simulink model "Quadcopter"  (R2022a)
settings: Solver=VariableStepAuto  StartTime=0.0  StopTime=10.0  RelTol=1e-3
settings Model: Creator=Erfan  LastModifiedBy=Erfan

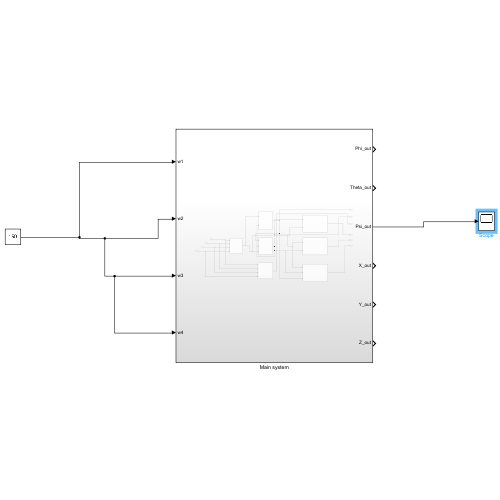
[thumbnail: Simulink's stored preview of the top-level diagram]
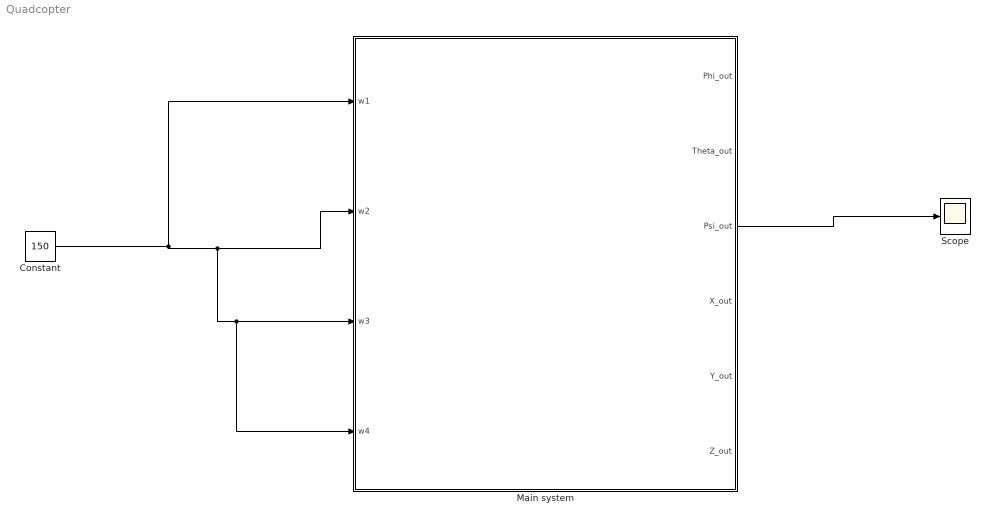
== system Quadcopter ==
  Constant : Constant  Value=150
  Main system : Subsystem
  Scope : Scope
  wires:
  Constant/1 -> Main system/4(w4), Main system/3(w3), Main system/2(w2), Main system/1(w1)
  Main system/3(Psi_out) -> Scope/1

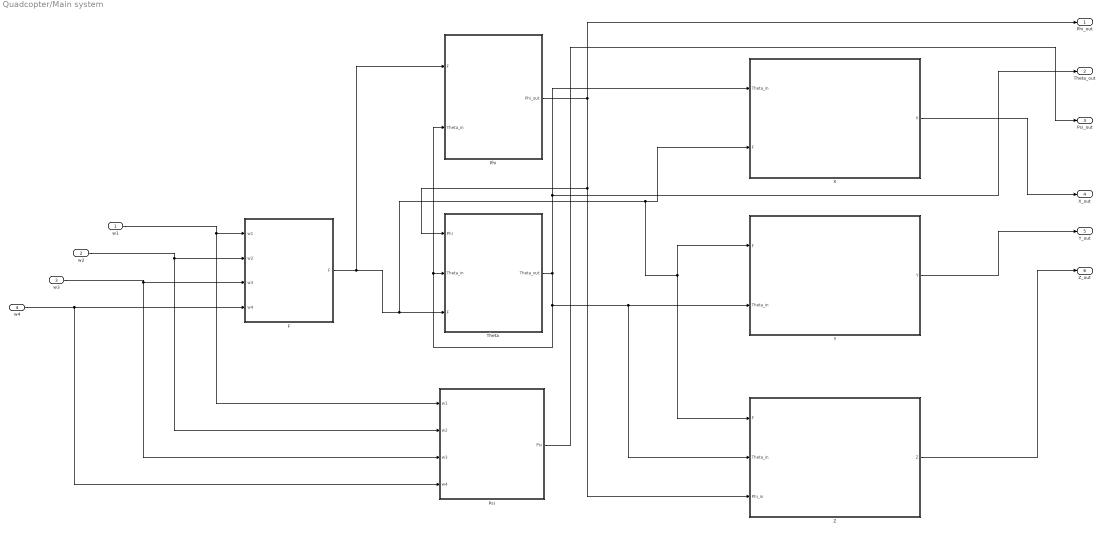
== system Quadcopter/Main system ==
  w1 : Inport
  w2 : Inport  Port=2
  w3 : Inport  Port=3
  w4 : Inport  Port=4
  F : Subsystem
  Phi : Subsystem
  Psi : Subsystem
  Theta : Subsystem
  X : Subsystem
  Y : Subsystem
  Z : Subsystem
  Phi_out : Outport
  Theta_out : Outport  Port=2
  Psi_out : Outport  Port=3
  X_out : Outport  Port=4
  Y_out : Outport  Port=5
  Z_out : Outport  Port=6
  wires:
  w1/1 -> Psi/1(w1), F/1(w1)
  w2/1 -> Psi/2(w2), F/2(w2)
  w3/1 -> Psi/3(w3), F/3(w3)
  w4/1 -> Psi/4(w4), F/4(w4)
  Phi/1(Phi_out) -> Phi_out/1, Theta/1(Phi), Z/3(Phi_in)
  F/1(F) -> Phi/1(F), Z/1(F), Y/1(F), X/2(F), Theta/3(F)
  Theta/1(Theta_out) -> Z/2(Theta_in), Y/2(Theta_in), Phi/2(Theta_in), Theta/2(Theta_in), Theta_out/1, X/1(Theta_in)
  X/1(X) -> X_out/1
  Psi/1(Psi) -> Psi_out/1
  Y/1(Y) -> Y_out/1
  Z/1(Z) -> Z_out/1

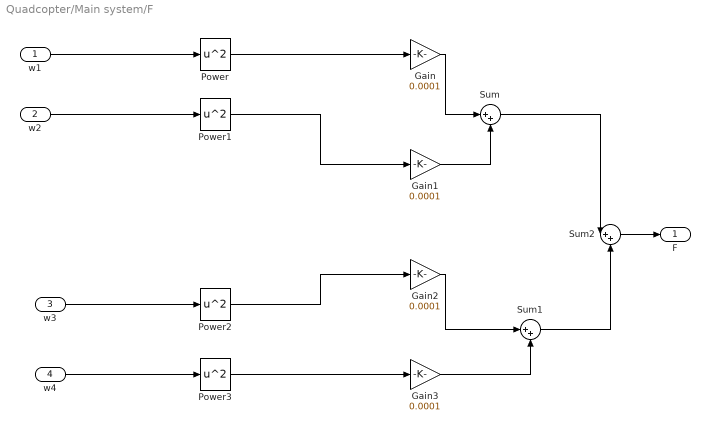
== system Quadcopter/Main system/F ==
  w1 : Inport
  w2 : Inport  Port=2
  w3 : Inport  Port=3
  w4 : Inport  Port=4
  Gain{,1..3} (4 alike) : Gain  Gain=0.0001
  Power{,1..3} (4 alike) : Math  Operator=square
  Sum : Sum  Inputs=|++
  Sum1 : Sum  Inputs=|++
  Sum2 : Sum  Inputs=|++
  F : Outport
  wires:
  Gain/1 -> Sum/1
  Sum2/1 -> F/1
  Power1/1 -> Gain1/1
  Sum/1 -> Sum2/1
  Sum1/1 -> Sum2/2
  Gain2/1 -> Sum1/1
  Power3/1 -> Gain3/1
  Gain3/1 -> Sum1/2
  Power/1 -> Gain/1
  w3/1 -> Power2/1
  w4/1 -> Power3/1
  Power2/1 -> Gain2/1
  Gain1/1 -> Sum/2
  w2/1 -> Power1/1
  w1/1 -> Power/1

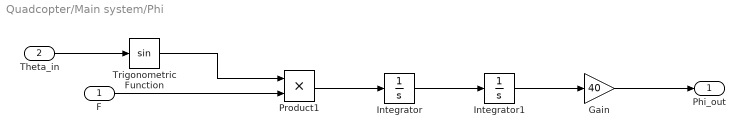
== system Quadcopter/Main system/Phi ==
  F : Inport
  Theta_in : Inport  Port=2
  Gain : Gain  Gain=40
  Integrator : Integrator
  Integrator1 : Integrator
  Product1 : Product
  Trigonometric Function : Trigonometry
  Phi_out : Outport
  wires:
  Integrator/1 -> Integrator1/1
  Gain/1 -> Phi_out/1
  Theta_in/1 -> Trigonometric Function/1
  Product1/1 -> Integrator/1
  Integrator1/1 -> Gain/1
  Trigonometric Function/1 -> Product1/1
  F/1 -> Product1/2

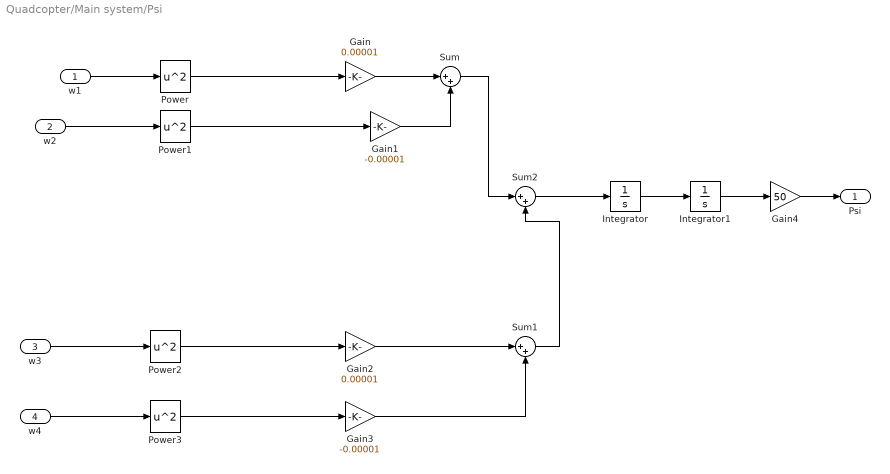
== system Quadcopter/Main system/Psi ==
  w1 : Inport
  w2 : Inport  Port=2
  w3 : Inport  Port=3
  w4 : Inport  Port=4
  Gain : Gain  Gain=0.00001
  Gain1 : Gain  Gain=-0.00001
  Gain2 : Gain  Gain=0.00001
  Gain3 : Gain  Gain=-0.00001
  Gain4 : Gain  Gain=50
  Integrator : Integrator
  Integrator1 : Integrator
  Power{,1..3} (4 alike) : Math  Operator=square
  Sum : Sum  Inputs=|++
  Sum1 : Sum  Inputs=|++
  Sum2 : Sum  Inputs=|++
  Psi : Outport
  wires:
  Power3/1 -> Gain3/1
  Power1/1 -> Gain1/1
  Gain4/1 -> Psi/1
  Gain2/1 -> Sum1/1
  Integrator1/1 -> Gain4/1
  Sum2/1 -> Integrator/1
  Sum1/1 -> Sum2/2
  Integrator/1 -> Integrator1/1
  Power/1 -> Gain/1
  Gain1/1 -> Sum/2
  Gain3/1 -> Sum1/2
  Power2/1 -> Gain2/1
  Sum/1 -> Sum2/1
  Gain/1 -> Sum/1
  w4/1 -> Power3/1
  w3/1 -> Power2/1
  w2/1 -> Power1/1
  w1/1 -> Power/1

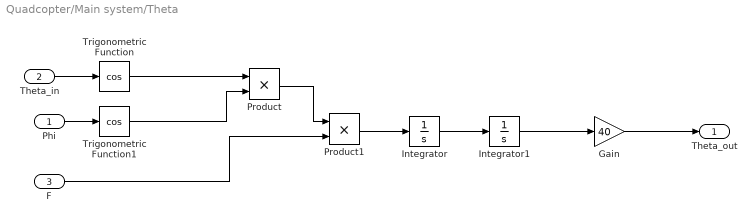
== system Quadcopter/Main system/Theta ==
  Phi : Inport
  Theta_in : Inport  Port=2
  F : Inport  Port=3
  Gain : Gain  Gain=40
  Integrator : Integrator
  Integrator1 : Integrator
  Product : Product
  Product1 : Product
  Trigonometric Function : Trigonometry  Operator=cos
  Trigonometric Function1 : Trigonometry  Operator=cos
  Theta_out : Outport
  wires:
  Integrator1/1 -> Gain/1
  Product1/1 -> Integrator/1
  Product/1 -> Product1/1
  Trigonometric Function1/1 -> Product/2
  Integrator/1 -> Integrator1/1
  Trigonometric Function/1 -> Product/1
  Gain/1 -> Theta_out/1
  Theta_in/1 -> Trigonometric Function/1
  Phi/1 -> Trigonometric Function1/1
  F/1 -> Product1/2

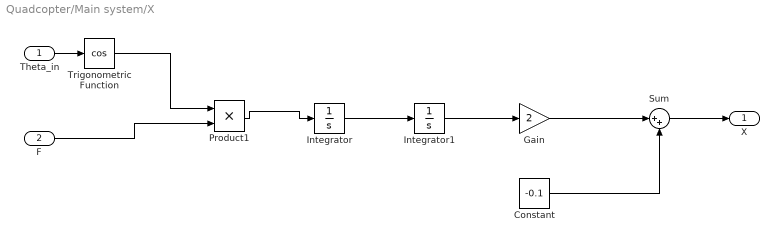
== system Quadcopter/Main system/X ==
  Theta_in : Inport
  F : Inport  Port=2
  Constant : Constant  Value=-0.1  SampleTime=-1
  Gain : Gain  Gain=2
  Integrator : Integrator
  Integrator1 : Integrator
  Product1 : Product
  Sum : Sum  Inputs=|++
  Trigonometric Function : Trigonometry  Operator=cos
  X : Outport
  wires:
  Sum/1 -> X/1
  Theta_in/1 -> Trigonometric Function/1
  Gain/1 -> Sum/1
  Integrator1/1 -> Gain/1
  Trigonometric Function/1 -> Product1/1
  Integrator/1 -> Integrator1/1
  Constant/1 -> Sum/2
  Product1/1 -> Integrator/1
  F/1 -> Product1/2

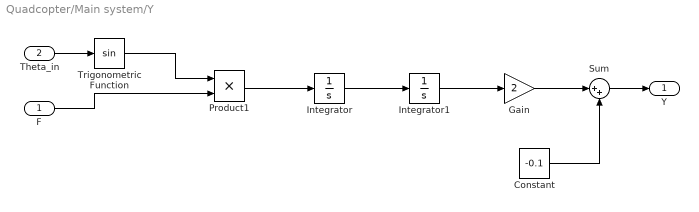
== system Quadcopter/Main system/Y ==
  F : Inport
  Theta_in : Inport  Port=2
  Constant : Constant  Value=-0.1  SampleTime=-1
  Gain : Gain  Gain=2
  Integrator : Integrator
  Integrator1 : Integrator
  Product1 : Product
  Sum : Sum  Inputs=|++
  Trigonometric Function : Trigonometry
  Y : Outport
  wires:
  Theta_in/1 -> Trigonometric Function/1
  Sum/1 -> Y/1
  Gain/1 -> Sum/1
  Integrator1/1 -> Gain/1
  Constant/1 -> Sum/2
  Integrator/1 -> Integrator1/1
  Product1/1 -> Integrator/1
  Trigonometric Function/1 -> Product1/1
  F/1 -> Product1/2

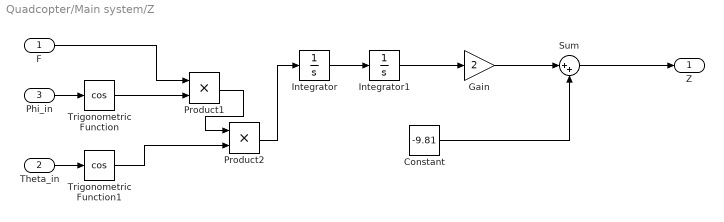
== system Quadcopter/Main system/Z ==
  F : Inport
  Theta_in : Inport  Port=2
  Phi_in : Inport  Port=3
  Constant : Constant  Value=-9.81  SampleTime=-1
  Gain : Gain  Gain=2
  Integrator : Integrator
  Integrator1 : Integrator
  Product1 : Product
  Product2 : Product
  Sum : Sum  Inputs=|++
  Trigonometric Function : Trigonometry  Operator=cos
  Trigonometric Function1 : Trigonometry  Operator=cos
  Z : Outport
  wires:
  Constant/1 -> Sum/2
  F/1 -> Product1/1
  Trigonometric Function/1 -> Product1/2
  Trigonometric Function1/1 -> Product2/2
  Product1/1 -> Product2/1
  Sum/1 -> Z/1
  Integrator1/1 -> Gain/1
  Gain/1 -> Sum/1
  Integrator/1 -> Integrator1/1
  Product2/1 -> Integrator/1
  Phi_in/1 -> Trigonometric Function/1
  Theta_in/1 -> Trigonometric Function1/1
